simulink model "PS84CL"  (Simulink 8.2)
settings: Solver=ode45  StartTime=0.0  StopTime=10.0  RelTol=1e-3
values from neighbouring files (symbols this model uses):
  P_den = [1 2 0]    [PS8_4.m]
  P_num = [1 -a]    [PS8_4.m]
undefined symbols (not defined in the file or in its folder): K_den, K_num
settings Model: Creator=Yili  LastModifiedBy=MQ
settings DataIOCC: SignalLoggingSaveFormat=Dataset
settings OptimizationCC: ExpressionDepthLimit=128
settings DebuggingCC: FcnCallInpInsideContextMsg=EnableAllAsError  StateNameClashWarn=none
settings GRTTargetCC: CombineOutputUpdateFcns=on  GRTInterface=off

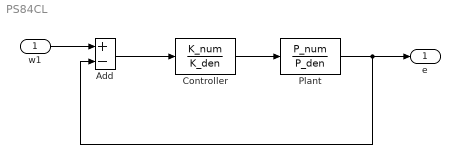
== system PS84CL ==
  w1 : Inport
  Add : Sum  Inputs=+-
  Controller : TransferFcn  Numerator=K_num  Denominator=K_den
  Plant : TransferFcn  Numerator=P_num  Denominator=P_den
  e : Outport
  wires:
  Controller/1 -> Plant/1
  Add/1 -> Controller/1
  Plant/1 -> e/1, Add/2
  w1/1 -> Add/1
